simulink model "model3robots"  (R2022a)
settings: Solver=VariableStepAuto  StartTime=0.0  StopTime=Inf  RelTol=1e-3
(part 1 of 2)
settings Model: Creator=mateu  LastModifiedBy=mateu

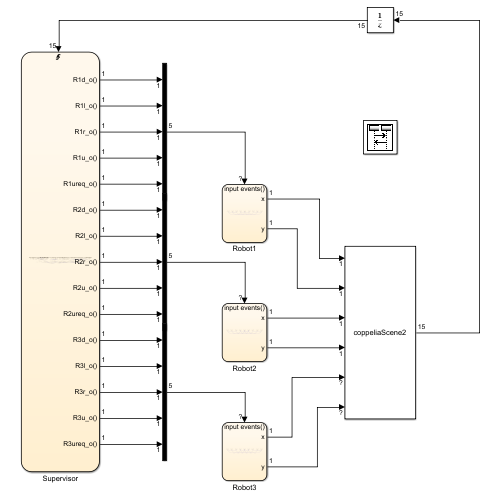
[thumbnail: Simulink's stored preview of the top-level diagram]
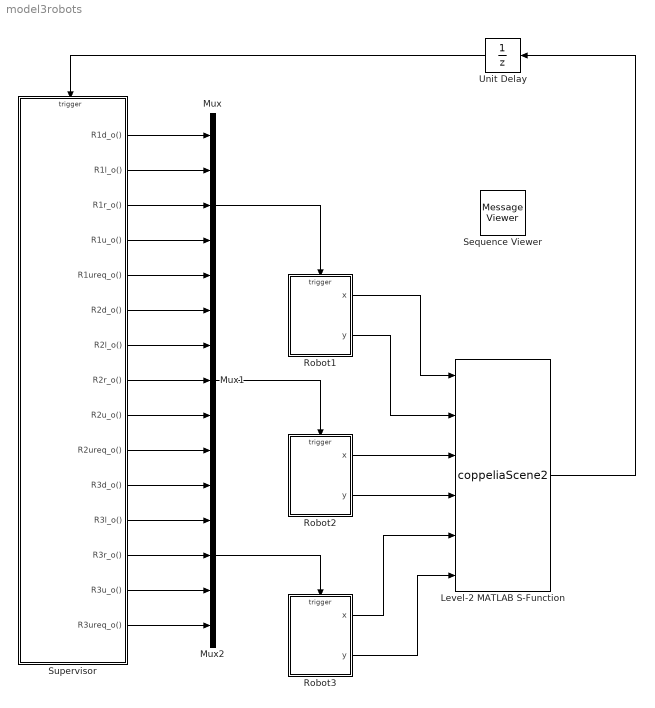
== system model3robots ==
  Level-2 MATLAB S-Function : M-S-Function  FunctionName=coppeliaScene2
  Mux : Mux  Inputs=5
  Mux1 : Mux  Inputs=5
  Mux2 : Mux  Inputs=5
  Robot1 : Stateflow chart  TreatAsAtomicUnit=on
  Robot2 : Stateflow chart  TreatAsAtomicUnit=on
  Robot3 : Stateflow chart  TreatAsAtomicUnit=on
  Sequence Viewer : MessageViewer
  Supervisor : Stateflow chart  TreatAsAtomicUnit=on
  Unit Delay : UnitDelay  SampleTime=-1  HasFrameUpgradeWarning=on
  wires:
  Level-2 MATLAB S-Function/1 -> Unit Delay/1
  Mux/1 -> Robot1/Trigger
  Mux1/1 -> Robot2/Trigger
  Mux2/1 -> Robot3/Trigger
  Robot1/1(x) -> Level-2 MATLAB S-Function/1
  Robot1/2(y) -> Level-2 MATLAB S-Function/2
  Robot2/1(x) -> Level-2 MATLAB S-Function/3
  Robot2/2(y) -> Level-2 MATLAB S-Function/4
  Robot3/1(x) -> Level-2 MATLAB S-Function/5
  Robot3/2(y) -> Level-2 MATLAB S-Function/6
  Supervisor/1(R1d_o()) -> Mux/1
  Supervisor/2(R1l_o()) -> Mux/2
  Supervisor/3(R1r_o()) -> Mux/3
  Supervisor/4(R1u_o()) -> Mux/4
  Supervisor/5(R1ureq_o()) -> Mux/5
  Supervisor/6(R2d_o()) -> Mux1/1
  Supervisor/7(R2l_o()) -> Mux1/2
  Supervisor/8(R2r_o()) -> Mux1/3
  Supervisor/9(R2u_o()) -> Mux1/4
  Supervisor/10(R2ureq_o()) -> Mux1/5
  Supervisor/11(R3d_o()) -> Mux2/1
  Supervisor/12(R3l_o()) -> Mux2/2
  Supervisor/13(R3r_o()) -> Mux2/3
  Supervisor/14(R3u_o()) -> Mux2/4
  Supervisor/15(R3ureq_o()) -> Mux2/5
  Unit Delay/1 -> Supervisor/Trigger

== stateflow chart model3robots/Robot2 ==
  settings: executeAtInitialization=1
  state s1
    x=1;
    y=1;
  state s2
    x=1;
    y=2;
  state s3
    x=1;
    y=3;
  state s4
    x=2;
    y=1;
  state s5
    x=2;
    y=2;
  state s6
    x=2;
    y=3;
  state s7
    x=3;
    y=1;
  state s8
    x=3;
    y=2;
  state s9
    x=3;
    y=3;
  (default) -> s4
  s2 -> s1 [order 1] : R2d
  s4 -> s1 [order 1] : R2l
  s1 -> s4 [order 1] : R2r
  s1 -> s2 [order 2] : R2u
  s3 -> s2 [order 1] : R2d
  s5 -> s2 [order 2] : R2l
  s2 -> s5 [order 2] : R2r
  s2 -> s3 [order 3] : R2u
  s6 -> s3 [order 2] : R2l
  s3 -> s6 [order 2] : R2r
  s5 -> s4 [order 1] : R2d
  s7 -> s4 [order 1] : R2l
  s4 -> s7 [order 2] : R2r
  s4 -> s5 [order 3] : R2u
  s6 -> s5 [order 1] : R2d
  s8 -> s5 [order 2] : R2l
  s5 -> s8 [order 3] : R2r
  s5 -> s6 [order 4] : R2u
  s5 -> s6 [order 5] : R2ureq
  s9 -> s6 [order 2] : R2l
  s6 -> s9 [order 3] : R2r
  s8 -> s7 [order 1] : R2d
  s7 -> s8 [order 2] : R2u
  s9 -> s8 [order 1] : R2d
  s8 -> s9 [order 3] : R2u
  data: x output double; y output double
  events: R2d input FUNCTION_CALL_EVENT; R2l input FUNCTION_CALL_EVENT; R2r input FUNCTION_CALL_EVENT; R2u input FUNCTION_CALL_EVENT; R2ureq input FUNCTION_CALL_EVENT

== stateflow chart model3robots/Robot3 ==
  settings: executeAtInitialization=1
  state s1
    x=1;
    y=1;
  state s2
    x=1;
    y=2;
  state s3
    x=1;
    y=3;
  state s4
    x=2;
    y=1;
  state s5
    x=2;
    y=2;
  state s6
    x=2;
    y=3;
  state s7
    x=3;
    y=1;
  state s8
    x=3;
    y=2;
  state s9
    x=3;
    y=3;
  (default) -> s7
  s2 -> s1 [order 1] : R3d
  s4 -> s1 [order 1] : R3l
  s1 -> s4 [order 1] : R3r
  s1 -> s2 [order 2] : R3u
  s3 -> s2 [order 1] : R3d
  s5 -> s2 [order 2] : R3l
  s2 -> s5 [order 2] : R3r
  s2 -> s3 [order 3] : R3u
  s6 -> s3 [order 2] : R3l
  s3 -> s6 [order 2] : R3r
  s5 -> s4 [order 1] : R3d
  s7 -> s4 [order 1] : R3l
  s4 -> s7 [order 2] : R3r
  s4 -> s5 [order 3] : R3u
  s6 -> s5 [order 1] : R3d
  s8 -> s5 [order 2] : R3l
  s5 -> s8 [order 3] : R3r
  s5 -> s6 [order 4] : R3u
  s9 -> s6 [order 2] : R3l
  s6 -> s9 [order 3] : R3r
  s8 -> s7 [order 1] : R3d
  s7 -> s8 [order 2] : R3u
  s9 -> s8 [order 1] : R3d
  s8 -> s9 [order 3] : R3u
  s8 -> s9 [order 4] : R3ureq
  data: x output double; y output double
  events: R3d input FUNCTION_CALL_EVENT; R3l input FUNCTION_CALL_EVENT; R3r input FUNCTION_CALL_EVENT; R3u input FUNCTION_CALL_EVENT; R3ureq input FUNCTION_CALL_EVENT

== stateflow chart model3robots/Robot1 ==
  settings: executeAtInitialization=1
  state s1
    x=1;
    y=1;
  state s2
    x=1;
    y=2;
  state s3
    x=1;
    y=3;
  state s4
    x=2;
    y=1;
  state s5
    x=2;
    y=2;
  state s6
    x=2;
    y=3;
  state s7
    x=3;
    y=1;
  state s8
    x=3;
    y=2;
  state s9
    x=3;
    y=3;
  (default) -> s1
  s2 -> s1 [order 1] : R1d
  s4 -> s1 [order 1] : R1l
  s1 -> s4 [order 1] : R1r
  s1 -> s2 [order 2] : R1u
  s3 -> s2 [order 1] : R1d
  s5 -> s2 [order 2] : R1l
  s2 -> s5 [order 2] : R1r
  s2 -> s3 [order 3] : R1u
  s2 -> s3 [order 4] : R1ureq
  s6 -> s3 [order 2] : R1l
  s3 -> s6 [order 2] : R1r
  s5 -> s4 [order 1] : R1d
  s7 -> s4 [order 1] : R1l
  s4 -> s7 [order 2] : R1r
  s4 -> s5 [order 3] : R1u
  s6 -> s5 [order 1] : R1d
  s8 -> s5 [order 2] : R1l
  s5 -> s8 [order 3] : R1r
  s5 -> s6 [order 4] : R1u
  s9 -> s6 [order 2] : R1l
  s6 -> s9 [order 3] : R1r
  s8 -> s7 [order 1] : R1d
  s7 -> s8 [order 2] : R1u
  s9 -> s8 [order 1] : R1d
  s8 -> s9 [order 3] : R1u
  data: x output double; y output double
  events: R1d input FUNCTION_CALL_EVENT; R1l input FUNCTION_CALL_EVENT; R1r input FUNCTION_CALL_EVENT; R1u input FUNCTION_CALL_EVENT; R1ureq input FUNCTION_CALL_EVENT
